simulink model "BlackStart"  (R2023a)
settings: Solver=FixedStepAuto  StartTime=0.0  StopTime=10.0  FixedStep=Ts  RelTol=1e-3
model mask{referenceFrequency=referenceFrequency, controllerBlackStart=controllerBlackStart, voltageLevel1=voltageLevel1, voltageLevel2=voltageLevel2, voltageLevel3=voltageLevel3, delayLevel1=delayLevel1, delayLevel2=delayLevel2, delayLevel3=delayLevel3}
  mask prompts: referenceFrequency "Reference Frequency"; controllerBlackStart "Black Start Time"; voltageLevel1 "Level1"; voltageLevel2 "Level2"; voltageLevel3 "Level3"; delayLevel1 "Delay1"; delayLevel2 "Delay2"; delayLevel3 "Delay3"
model workspace (MAT data in the model file):
  Ts = 0.001
  controllerBlackStart = 0
  delayLevel1 = 0
  delayLevel2 = 0
  delayLevel3 = 0
  referenceFrequency = 0
  voltageLevel1 = 0
  voltageLevel2 = 0
  voltageLevel3 = 0
settings Model: ParameterArgumentNames=controllerBlackStart,delayLevel1,delayLevel2,delayLevel3,referenceFrequency,voltageLevel1,voltageLevel2,voltageLevel3  Creator=skota  LastModifiedBy=skota
settings DataIOCC: SaveFormat=StructureWithTime

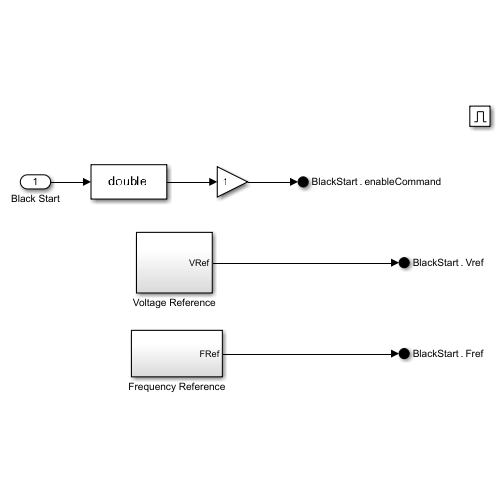
[thumbnail: Simulink's stored preview of the top-level diagram]
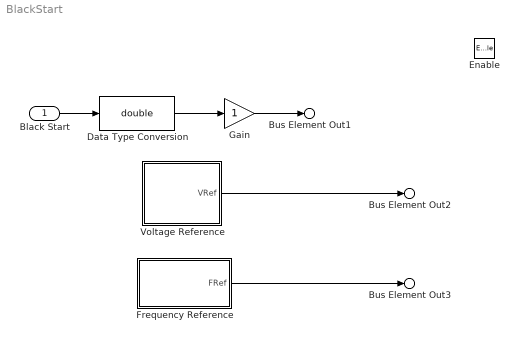
== system BlackStart ==
  Black Start : Inport  OutDataTypeStr=boolean
  Enable : EnablePort  OutDataTypeStr=boolean
  Data Type Conversion : DataTypeConversion  OutDataTypeStr=double  SaturateOnIntegerOverflow=off  RndMeth=Floor
  Frequency Reference : Subsystem
  Gain : Gain
  Voltage Reference : Subsystem
  Bus Element Out2 : Outport  PortName=BlackStart  Element=Vref
  Bus Element Out3 : Outport  PortName=BlackStart  Element=Fref
  Bus Element Out1 : Outport  PortName=BlackStart  Element=enableCommand
  wires:
  Gain/1 -> Bus Element Out1/1
  Black Start/1 -> Data Type Conversion/1
  Voltage Reference/1(VRef) -> Bus Element Out2/1
  Frequency Reference/1(FRef) -> Bus Element Out3/1
  Data Type Conversion/1 -> Gain/1

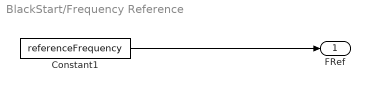
== system BlackStart/Frequency Reference ==
  Constant1 : Constant  Value=referenceFrequency
  FRef : Outport
  wires:
  Constant1/1 -> FRef/1

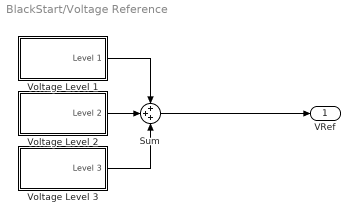
== system BlackStart/Voltage Reference ==
  Sum : Sum  Inputs=+++
  Voltage Level 1 : Subsystem
  Voltage Level 2 : Subsystem
  Voltage Level 3 : Subsystem
  VRef : Outport
  wires:
  Sum/1 -> VRef/1
  Voltage Level 2/1(Level 2) -> Sum/2
  Voltage Level 3/1(Level 3) -> Sum/3
  Voltage Level 1/1(Level 1) -> Sum/1

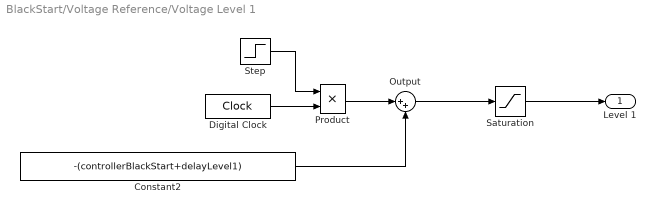
== system BlackStart/Voltage Reference/Voltage Level 1 ==
  Constant2 : Constant  DisableCoverage=on  Value=-(controllerBlackStart+delayLevel1)  OutDataTypeStr=Inherit: Inherit via back propagation  SampleTime=Ts
  Digital Clock : DigitalClock  SampleTime=Ts
  Output : Sum  Inputs=|++  InputSameDT=on  SaturateOnIntegerOverflow=on  OutDataTypeStr=Inherit: Same as first input
  Product : Product  DisableCoverage=on  InputSameDT=on  SaturateOnIntegerOverflow=on  OutDataTypeStr=Inherit: Same as first input
  Saturation : Saturate  UpperLimit=voltageLevel1  LowerLimit=0
  Step : Step  DisableCoverage=on  Time=controllerBlackStart+delayLevel1  OutDataTypeStr=fixdt('double', 'DataTypeOverride', 'Off')  SampleTime=Ts
  Level 1 : Outport
  wires:
  Digital Clock/1 -> Product/2
  Constant2/1 -> Output/2
  Saturation/1 -> Level 1/1
  Product/1 -> Output/1
  Output/1 -> Saturation/1
  Step/1 -> Product/1

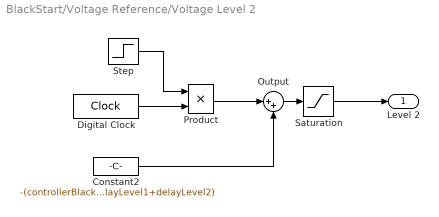
== system BlackStart/Voltage Reference/Voltage Level 2 ==
  Constant2 : Constant  DisableCoverage=on  Value=-(controllerBlackStart+delayLevel1+delayLevel2)  OutDataTypeStr=Inherit: Inherit via back propagation  SampleTime=Ts
  Digital Clock : DigitalClock  SampleTime=Ts
  Output : Sum  Inputs=|++  InputSameDT=on  SaturateOnIntegerOverflow=on  OutDataTypeStr=Inherit: Same as first input
  Product : Product  DisableCoverage=on  InputSameDT=on  SaturateOnIntegerOverflow=on  OutDataTypeStr=Inherit: Same as first input
  Saturation : Saturate  UpperLimit=voltageLevel2  LowerLimit=0
  Step : Step  DisableCoverage=on  Time=controllerBlackStart+delayLevel1+delayLevel2  OutDataTypeStr=fixdt('double', 'DataTypeOverride', 'Off')  SampleTime=Ts
  Level 2 : Outport
  wires:
  Step/1 -> Product/1
  Output/1 -> Saturation/1
  Product/1 -> Output/1
  Saturation/1 -> Level 2/1
  Constant2/1 -> Output/2
  Digital Clock/1 -> Product/2

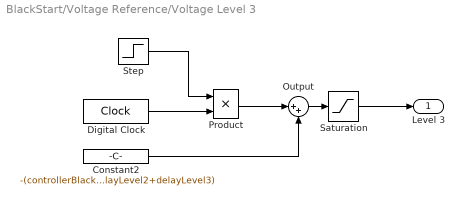
== system BlackStart/Voltage Reference/Voltage Level 3 ==
  Constant2 : Constant  DisableCoverage=on  Value=-(controllerBlackStart+delayLevel1+delayLevel2+delayLevel3)  OutDataTypeStr=Inherit: Inherit via back propagation  SampleTime=Ts
  Digital Clock : DigitalClock  SampleTime=Ts
  Output : Sum  Inputs=|++  InputSameDT=on  SaturateOnIntegerOverflow=on  OutDataTypeStr=Inherit: Same as first input
  Product : Product  DisableCoverage=on  InputSameDT=on  SaturateOnIntegerOverflow=on  OutDataTypeStr=Inherit: Same as first input
  Saturation : Saturate  UpperLimit=voltageLevel3  LowerLimit=0
  Step : Step  DisableCoverage=on  Time=controllerBlackStart+delayLevel1+delayLevel2+delayLevel3  OutDataTypeStr=fixdt('double', 'DataTypeOverride', 'Off')  SampleTime=Ts
  Level 3 : Outport
  wires:
  Digital Clock/1 -> Product/2
  Constant2/1 -> Output/2
  Saturation/1 -> Level 3/1
  Product/1 -> Output/1
  Output/1 -> Saturation/1
  Step/1 -> Product/1
